simulink model "AirStat"  (R2025b)
settings: Solver=VariableStepAuto  StartTime=0.0  StopTime=10  RelTol=1e-3
model workspace (MAT data in the model file):
  x1 = [0.6667 0.6087 1]
undefined symbols (not defined in the file): torch
libraries: pycoexlib x1
settings Model: Creator=acer  LastModifiedBy=acer

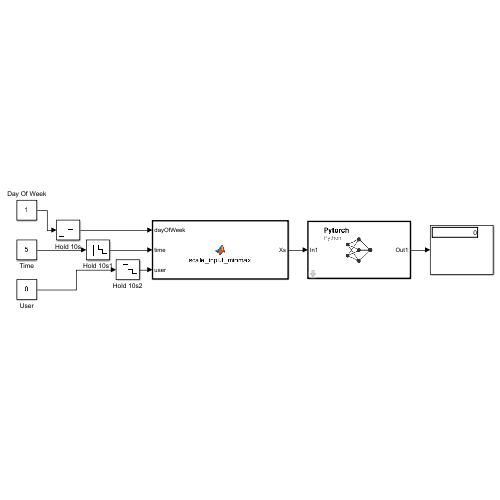
[thumbnail: Simulink's stored preview of the top-level diagram]
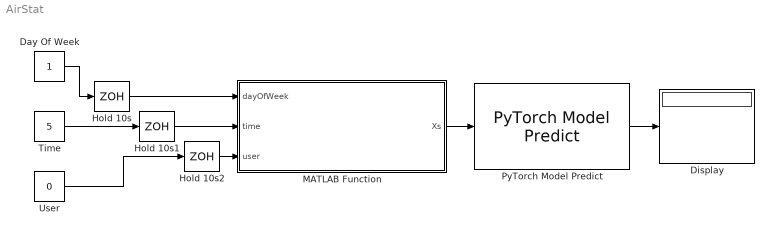
== system AirStat ==
  Day Of Week : Constant
  Display : Display
  Hold 10s : ZeroOrderHold  SampleTime=10
  Hold 10s1 : ZeroOrderHold  SampleTime=10
  Hold 10s2 : ZeroOrderHold  SampleTime=10
  MATLAB Function : MATLAB Function  TreatAsAtomicUnit=on
  PyTorch Model Predict : pycoexlib/PyTorch Model Predict  ModelFile=D:\Senior Jec\V1_Air_Controller_for_Simulink_ArgMax.pt  LoadCommandPopup=torch.load()  DeviceComboBox=cpu  InputTable={ 'In1', 'float32', '', '' }  OutputTable={ 'Out1', '', '' }  SampleTime=-1  TorchLoadCommand=torch.load()  Device=cpu  InputDatatypes=float32  InputPermutations=[]  OutputPermutations=[]  PythonCoexecutionBlockType=PyTorchModelBlock  VariableOutputMaxSizes=[]
  Time : Constant  Value=5
  User : Constant  Value=0
  wires:
  PyTorch Model Predict/1 -> Display/1
  Time/1 -> Hold 10s1/1
  User/1 -> Hold 10s2/1
  Day Of Week/1 -> Hold 10s/1
  MATLAB Function/1(Xs) -> PyTorch Model Predict/1
  Hold 10s/1 -> MATLAB Function/1(dayOfWeek)
  Hold 10s1/1 -> MATLAB Function/2(time)
  Hold 10s2/1 -> MATLAB Function/3(user)

== matlab function AirStat/MATLAB Function ==
  data: dayOfWeek input; Xs output; time input; user input
function Xs = scale_input_minmax(dayOfWeek, time, user)

    % ---- ใส่ค่า Min / Max ตรงนี้ ----
    data_min = [1 0 0];      % จาก sklearn MinMaxScaler
    data_max = [7 23 60];

    % รวมอินพุตเป็น Row Vector 1×3
    X = [dayOfWeek, time, user];
    X = reshape(X, 1, 3);    % ป้องกันกลายเป็น 3×3

    % Min-Max Scaling
    Xs = (X - data_min) ./ (data_max - data_min);

end
